simulink model "Heat_exchanger_model"  (R2016a)
settings: Solver=VariableStepAuto  StartTime=0.0  StopTime=450  FixedStep=0.0001  RelTol=1e-3  AbsTol=1e-3
libraries: simulink x1
settings Model: Creator=EBUKA  LastModifiedBy=EBUKA
settings SolverCC: AlgebraicLoopSolver=LineSearch
settings GRTTargetCC: GeneratePreprocessorConditionals=Use local settings
settings SimscapeCC: SimscapeLogType=all  SimscapeLogDataHistory=10000

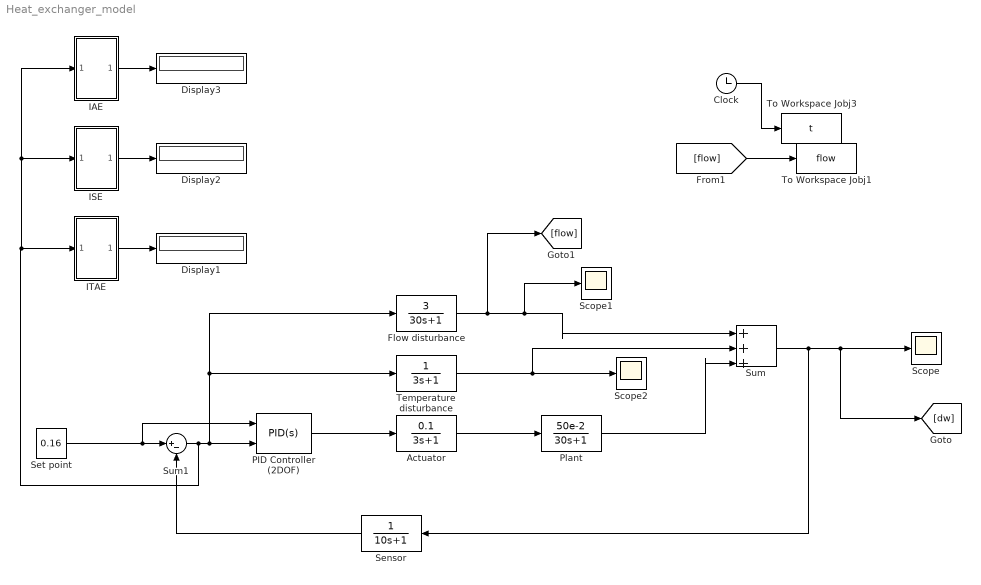
== system Heat_exchanger_model ==
  Actuator : TransferFcn  Numerator=[0.1]  Denominator=[3 1]
  Clock : Clock
  Display1 : Display
  Display2 : Display
  Display3 : Display
  Flow disturbance : TransferFcn  Numerator=[3]  Denominator=[30 1]
  IAE : Subsystem
  ISE : Subsystem
  ITAE : Subsystem
  PID Controller (2DOF) : simulink/Continuous/PID Controller (2DOF)  Controller=PID  TimeDomain=Continuous-time  SampleTime=-1  IntegratorMethod=Forward Euler  FilterMethod=Forward Euler  Form=Parallel  UseFilter=on  ControllerParametersSource=internal  P=-189.2859  I=-14.3812  D=-558.2981  N=16.8029  b=0.0227  c=0.0748  InitialConditionSource=internal  InitialConditionForIntegrator=0  InitialConditionForFilter=0  ExternalReset=none  LimitOutput=off  UpperSaturationLimit=inf  LowerSaturationLimit=-inf  LinearizeAsGain=on  AntiWindupMode=none  Kb=1  TrackingMode=off  Kt=1  PParamMin=[]  PParamMax=[]  IParamMin=[]  IParamMax=[]  DParamMin=[]  DParamMax=[]  NParamMin=[]  NParamMax=[]  bParamMin=[]  bParamMax=[]  cParamMin=[]  cParamMax=[]  KbParamMin=[]  KbParamMax=[]  KtParamMin=[]  KtParamMax=[]  POutMin=[]  POutMax=[]  IOutMin=[]  IOutMax=[]  DOutMin=[]  DOutMax=[]  NOutMin=[]  NOutMax=[]  bOutMin=[]  bOutMax=[]  cOutMin=[]  cOutMax=[]  KbOutMin=[]  KbOutMax=[]  KtOutMin=[]  KtOutMax=[]  IntegratorOutMin=[]  IntegratorOutMax=[]  FilterOutMin=[]  FilterOutMax=[]  SumOutMin=[]  SumOutMax=[]  Sum1OutMin=[]  Sum1OutMax=[]  Sum2OutMin=[]  Sum2OutMax=[]  Sum3OutMin=[]  Sum3OutMax=[]  SumI1OutMin=[]  SumI1OutMax=[]  SumI2OutMin=[]  SumI2OutMax=[]  SumI3OutMin=[]  SumI3OutMax=[]  SumDOutMin=[]  SumDOutMax=[]  SaturationOutMin=[]  SaturationOutMax=[]  IntegratorContinuousStateAttributes=''  IntegratorStateMustResolveToSignalObject=off  IntegratorRTWStateStorageClass=Auto  FilterContinuousStateAttributes=''  FilterStateMustResolveToSignalObject=off  FilterRTWStateStorageClass=Auto  DifferentiatorICPrevScaledInput=0  DifferentiatorOutMin=[]  DifferentiatorOutMax=[]
  Plant : TransferFcn  Numerator=[50e-2]  Denominator=[30 1]
  Scope : Scope
  Scope1 : Scope
  Scope2 : Scope
  Sensor : TransferFcn  Denominator=[10 1]
  Set point : Constant  Value=0.16
  Sum : Sum  Inputs=|+|+|+
  Sum1 : Sum  Inputs=|+-
  Temperature disturbance : TransferFcn  Denominator=[3 1]
  To Workspace Jobj1 : ToWorkspace  VariableName=flow  SampleTime=-1
  To Workspace Jobj3 : ToWorkspace  VariableName=t  SampleTime=-1
  wires:
  Temperature disturbance/1 -> Sum/2, Scope2/1
  Plant/1 -> Sum/3
  Actuator/1 -> Plant/1
  Sensor/1 -> Sum1/2
  Sum/1 -> [dw], Scope/1, Sensor/1
  Clock/1 -> To Workspace Jobj3/1
  [flow] -> To Workspace Jobj1/1
  Flow disturbance/1 -> [flow], Scope1/1, Sum/1
  Set point/1 -> PID Controller (2DOF)/1, Sum1/1
  PID Controller (2DOF)/1 -> Actuator/1
  Sum1/1 -> ISE/1(In1), IAE/1(In1), ITAE/1(In1), Flow disturbance/1, Temperature disturbance/1, PID Controller (2DOF)/2
  ITAE/1(Out1) -> Display1/1
  ISE/1(Out1) -> Display2/1
  IAE/1(Out1) -> Display3/1

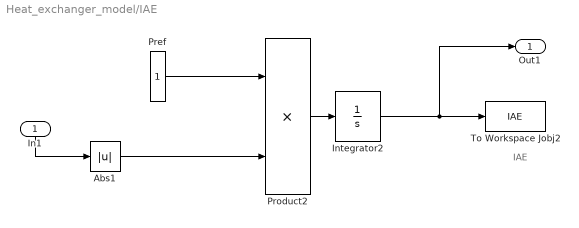
== system Heat_exchanger_model/IAE ==
  note: IAE
  In1 : Inport
  Abs1 : Abs
  Integrator2 : Integrator
  Pref : Constant
  Product2 : Product
  To Workspace Jobj2 : ToWorkspace  VariableName=IAE  SampleTime=-1
  Out1 : Outport
  wires:
  Product2/1 -> Integrator2/1
  Abs1/1 -> Product2/2
  In1/1 -> Abs1/1
  Integrator2/1 -> Out1/1, To Workspace Jobj2/1
  Pref/1 -> Product2/1

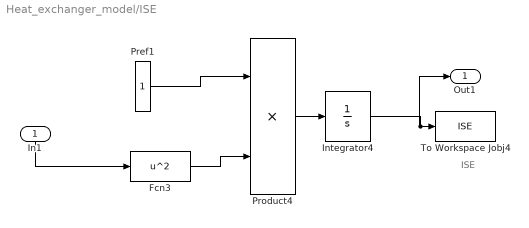
== system Heat_exchanger_model/ISE ==
  note: ISE
  In1 : Inport
  Fcn3 : Fcn  Expr=u^2
  Integrator4 : Integrator
  Pref1 : Constant
  Product4 : Product
  To Workspace Jobj4 : ToWorkspace  VariableName=ISE  SampleTime=-1
  Out1 : Outport
  wires:
  Pref1/1 -> Product4/1
  Integrator4/1 -> Out1/1, To Workspace Jobj4/1
  In1/1 -> Fcn3/1
  Product4/1 -> Integrator4/1
  Fcn3/1 -> Product4/2

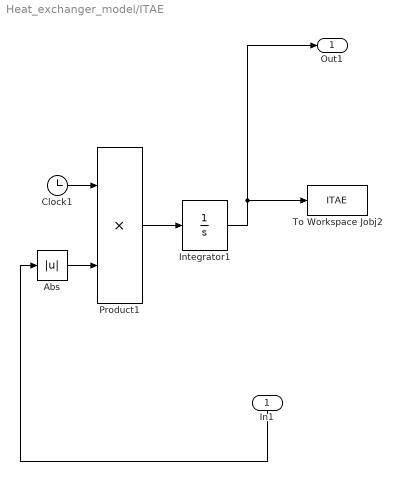
== system Heat_exchanger_model/ITAE ==
  In1 : Inport
  Abs : Abs
  Clock1 : Clock
  Integrator1 : Integrator
  Product1 : Product
  To Workspace Jobj2 : ToWorkspace  VariableName=ITAE  SampleTime=-1
  Out1 : Outport
  wires:
  In1/1 -> Abs/1
  Integrator1/1 -> Out1/1, To Workspace Jobj2/1
  Clock1/1 -> Product1/1
  Abs/1 -> Product1/2
  Product1/1 -> Integrator1/1
